simulink model "sinx"  (R2021b)
settings: Solver=ode5  StartTime=0.0  StopTime=2*pi  FixedStep=0.01  RelTol=1e-3
settings Model: Creator=86195  LastModifiedBy=86195

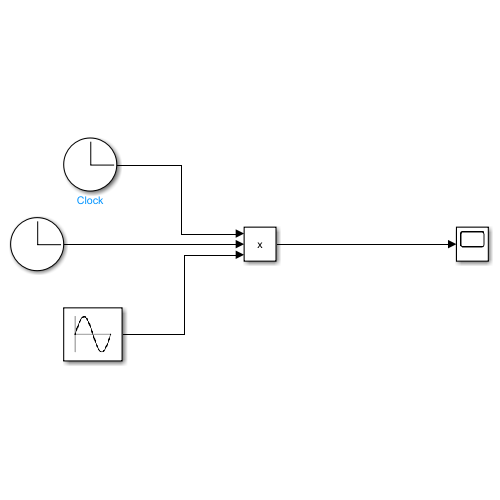
[thumbnail: Simulink's stored preview of the top-level diagram]
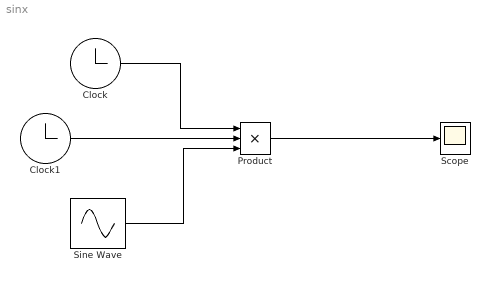
== system sinx ==
  Clock : Clock
  Clock1 : Clock
  Product : Product  Inputs=3
  Scope : Scope
  Sine Wave : Sin  Frequency=2*pi  SampleTime=0
  wires:
  Clock/1 -> Product/1
  Sine Wave/1 -> Product/3
  Clock1/1 -> Product/2
  Product/1 -> Scope/1
